simulink subsystem "Auto_FF_Scale_Processor"  (R2023a)
settings: Solver=VariableStepAuto  StartTime=0.0  StopTime=10.0  RelTol=1e-3
undefined symbols (not defined in the file or in its folder): angular, linear
libraries: ros2lib x4
settings Model: Creator=hollis  LastModifiedBy=john

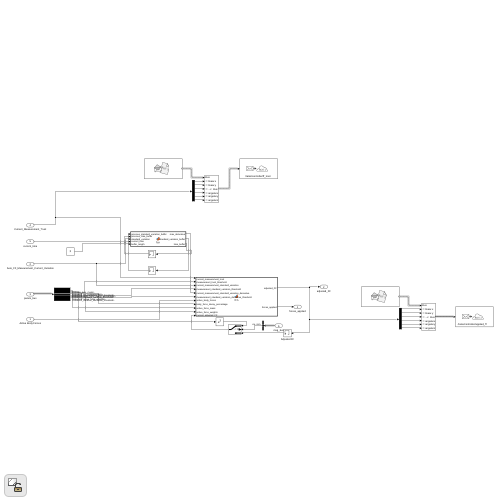
[thumbnail: Simulink's stored preview of the top-level diagram]
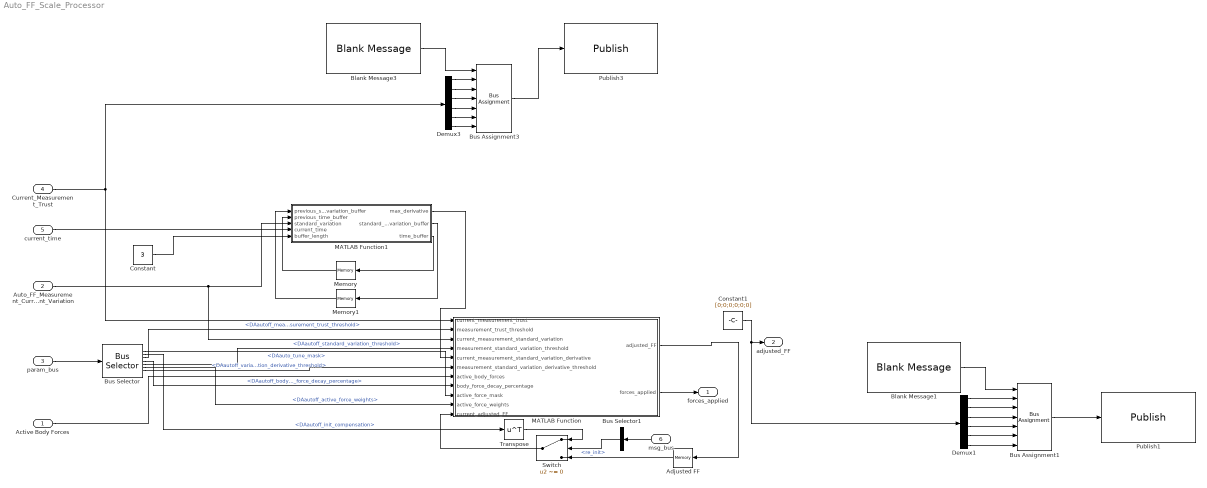
== system Auto_FF_Scale_Processor ==
  Active Body Forces : Inport
  Auto_FF_Measurement_Current_Variation : Inport  Port=2
  param_bus : Inport  Port=3
  Current_Measurement_Trust : Inport  Port=4
  current_time : Inport  Port=5
  msg_bus : Inport  Port=6
  Adjusted FF : Memory  InitialCondition=[0,0,0,0,0,0]'
  Blank Message1 : ros2lib/Blank Message  messageClass=Message  entityType=geometry_msgs/Twist  messageType=geometry_msgs/Twist  SampleTime=inf
  Blank Message3 : ros2lib/Blank Message  messageClass=Message  entityType=geometry_msgs/Twist  messageType=geometry_msgs/Twist  SampleTime=inf
  Bus Assignment1 : BusAssignment  AssignedSignals=linear.x,linear.y,linear.z,angular.x,angular.y,angular.z
  Bus Assignment3 : BusAssignment  AssignedSignals=linear.x,linear.y,linear.z,angular.x,angular.y,angular.z
  Bus Selector : BusSelector  OutputSignals=DAauto_tune_mask,DAautoff_init_compensation,DAautoff_measurement_trust_threshold,DAautoff_body_force_decay_percentage,DAautoff_standard_variation_threshold,DAautoff_active_force_weights,DAautoff_variation_derivative_threshold
  Bus Selector1 : BusSelector  OutputSignals=re_init
  Constant : Constant  Value=3
  Constant1 : Constant  Value=[0;0;0;0;0;0]
  Demux1 : Demux  Outputs=6
  Demux3 : Demux  Outputs=6
  MATLAB Function : MATLAB Function  TreatAsAtomicUnit=on
  MATLAB Function1 : MATLAB Function  TreatAsAtomicUnit=on
  Memory : Memory  InitialCondition=zeros(256,1)
  Memory1 : Memory  InitialCondition=zeros(256,6)
  Publish1 : ros2lib/Publish  topicSource=Specify your own  topic=/mercury/controller/applied_ff  messageType=geometry_msgs/Twist  QOSHistory=Keep last  QOSDepth=1  QOSReliability=Reliable  QOSDurability=Volatile
  Publish3 : ros2lib/Publish  topicSource=Specify your own  topic=/mercury/controller/ff_trust  messageType=geometry_msgs/Twist  QOSHistory=Keep last  QOSDepth=1  QOSReliability=Reliable  QOSDurability=Volatile
  Switch : Switch  Criteria=u2 ~= 0  SaturateOnIntegerOverflow=off  InputSameDT=off
  Transpose : Math  Operator=transpose
  forces_applied : Outport  OutDataTypeStr=boolean
  adjusted_FF : Outport  Port=2
  wires:
  MATLAB Function/2(forces_applied) -> forces_applied/1
  Current_Measurement_Trust/1 -> MATLAB Function/1(current_measurement_trust), Demux3/1
  param_bus/1 -> Bus Selector/1
  Bus Selector/1 -> MATLAB Function/9(active_force_mask)  "<DAauto_tune_mask>"
  Bus Selector/3 -> MATLAB Function/2(measurement_trust_threshold)  "<DAautoff_measurement_trust_threshold>"
  Bus Selector/4 -> MATLAB Function/8(body_force_decay_percentage)  "<DAautoff_body_force_decay_percentage>"
  Bus Selector/5 -> MATLAB Function/4(measurement_standard_variation_threshold)  "<DAautoff_standard_variation_threshold>"
  Bus Selector/6 -> MATLAB Function/10(active_force_weights)  "<DAautoff_active_force_weights>"
  Constant/1 -> MATLAB Function1/5(buffer_length)
  current_time/1 -> MATLAB Function1/4(current_time)
  Memory/1 -> MATLAB Function1/2(previous_time_buffer)
  Memory1/1 -> MATLAB Function1/1(previous_standard_variation_buffer)
  MATLAB Function1/3(time_buffer) -> Memory/1
  MATLAB Function1/2(standard_variation_buffer) -> Memory1/1
  Bus Selector/7 -> MATLAB Function/6(measurement_standard_variation_derivative_threshold)  "<DAautoff_variation_derivative_threshold>"
  Demux1/2 -> Bus Assignment1/3
  Demux1/1 -> Bus Assignment1/2
  Demux1/6 -> Bus Assignment1/7
  Demux1/5 -> Bus Assignment1/6
  Demux1/3 -> Bus Assignment1/4
  Blank Message1/1 -> Bus Assignment1/1
  Demux1/4 -> Bus Assignment1/5
  Bus Assignment1/1 -> Publish1/1
  MATLAB Function/1(adjusted_FF) -> Adjusted FF/1
  Auto_FF_Measurement_Current_Variation/1 -> MATLAB Function1/3(standard_variation), MATLAB Function/3(current_measurement_standard_variation)
  Demux3/1 -> Bus Assignment3/2
  Blank Message3/1 -> Bus Assignment3/1
  Demux3/2 -> Bus Assignment3/3
  Demux3/3 -> Bus Assignment3/4
  Demux3/4 -> Bus Assignment3/5
  Demux3/5 -> Bus Assignment3/6
  Demux3/6 -> Bus Assignment3/7
  Bus Assignment3/1 -> Publish3/1
  Active Body Forces/1 -> MATLAB Function/7(active_body_forces)
  MATLAB Function1/1(max_derivative) -> MATLAB Function/5(current_measurement_standard_variation_derivative)
  Switch/1 -> MATLAB Function/11(current_adjusted_FF)
  Adjusted FF/1 -> Switch/3
  msg_bus/1 -> Bus Selector1/1
  Bus Selector1/1 -> Switch/2  "<re_init>"
  Bus Selector/2 -> Transpose/1  "<DAautoff_init_compensation>"
  Transpose/1 -> Switch/1
  Constant1/1 -> adjusted_FF/1, Demux1/1

== matlab function Auto_FF_Scale_Processor/MATLAB Function ==
  data: current_measurement_trust input; adjusted_FF output; measurement_trust_threshold input; current_measurement_standard_variation input; measurement_standard_variation_threshold input; current_measurement_standard_variation_derivative input; measurement_standard_variation_derivative_threshold input; active_body_forces input; body_force_decay_percentage input; active_force_mask input; active_force_weights input; current_adjusted_FF input; forces_applied output
function [adjusted_FF, forces_applied] = fcn(current_measurement_trust, measurement_trust_threshold, current_measurement_standard_variation, measurement_standard_variation_threshold, current_measurement_standard_variation_derivative, measurement_standard_variation_derivative_threshold, active_body_forces, body_force_decay_percentage, active_force_mask, active_force_weights, current_adjusted_FF)

%determine if the axis meets the trust requirement
trust_mask = current_measurement_trust' > measurement_trust_threshold;

%detmerine if the axis meets the standard variation requirement
standard_variation_mask = current_measurement_standard_variation' < measurement_standard_variation_threshold;

derivative_mask = current_measurement_standard_variation_derivative < measurement_standard_variation_derivative_threshold;

%determine if the axis is ready for convergence
overall_mask = active_force_mask .* standard_variation_mask .* trust_mask .* derivative_mask;

%default setup
adjusted_FF = current_adjusted_FF;
forces_applied = false;

if(sum(overall_mask) >= 1)

    %determine the target axis - currently pull the axis with the largest
    %weighted active force 
    [max_masked, max_axis_masked] = max(abs(active_force_weights .* overall_mask .* active_body_forces'));
    [max_val, max_axis] = max(abs(active_force_weights .* active_force_mask .* active_body_forces'));

    %if the max axis is not the axis of most concern
    if(max_axis ~= max_axis_masked)
        if(max_val > max_masked)
            return
        end
    end

    %calulate the active force decay factor - only one non-zero term
    body_force_decay_percentage_masked = zeros([6,1]);
    body_force_decay_percentage_masked(max_axis) = body_force_decay_percentage(max_axis);

    %calculate the force to apply to the auto FF
    delta_FF = body_force_decay_percentage_masked .* active_body_forces;
    
    adjusted_FF = current_adjusted_FF + delta_FF;
    forces_applied = true;


end

== matlab function Auto_FF_Scale_Processor/MATLAB Function1 ==
  data: previous_standard_variation_buffer input; max_derivative output; previous_time_buffer input; standard_variation input; current_time input; buffer_length input; standard_variation_buffer output; time_buffer output
function [max_derivative, standard_variation_buffer, time_buffer] = fcn(previous_standard_variation_buffer, previous_time_buffer, standard_variation, current_time, buffer_length)

end_found = false;
end_index = 0;
while(end_found == false)

    end_index = end_index + 1;

    if(current_time - previous_time_buffer > buffer_length)
        end_found = true;
    end

    if(end_index == 256)
        end_found = true;
    end
end

time_buffer = zeros(256,1);
standard_variation_buffer = zeros(256,6);
time_buffer(2:256) = previous_time_buffer(1:255);
time_buffer(1) = current_time;
standard_variation_buffer(2:256,:) = previous_standard_variation_buffer(1:255, :);
standard_variation_buffer(1, :) = standard_variation;

if(end_index == 1)
    max_derivative = [1000,1000,1000,1000,1000,1000];

    return
end

derivatives = zeros(end_index - 1,6);
for i = 1:(end_index - 1)
    derivatives(i, :) = (previous_standard_variation_buffer(i,:) - previous_standard_variation_buffer(i+1,:)) ./ (previous_time_buffer(i) - previous_time_buffer(i+1));
end

max_derivative = max(abs(derivatives), [], 1);
